simulink model "gm_model_biquad_wfa"  (R2020b)
settings: Solver=VariableStepAuto  StartTime=0.0  StopTime=1  RelTol=1e-3
undefined symbols (not defined in the file or in its folder): dfilt, in_cos, Wkn
libraries: simulink x2, dsparch4 x1
settings Model: Creator=pablo  LastModifiedBy=pablo
settings OptimizationCC: BlockReduction=off  ConditionallyExecuteInputs=off
settings DebuggingCC: ArtificialAlgebraicLoopMsg=none  InheritedTsInSrcMsg=none

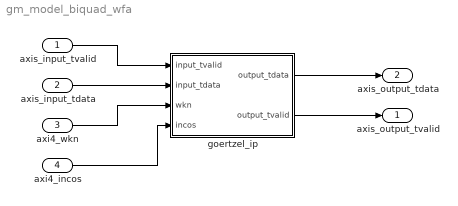
== system gm_model_biquad_wfa ==
  axis_input_tvalid : Inport  OutDataTypeStr=boolean  PortDimensions=1  SampleTime=0.001
  axis_input_tdata : Inport  Port=2  OutDataTypeStr=fixdt(1, 32, 16)  PortDimensions=1  SampleTime=0.001
  axi4_wkn : Inport  Port=3  OutDataTypeStr=fixdt(1, 32, 16)  PortDimensions=1  SampleTime=0.001
  axi4_incos : Inport  Port=4  OutDataTypeStr=fixdt(1, 32, 16)  PortDimensions=1  SampleTime=0.001
  goertzel_ip : Subsystem
  axis_output_tvalid : Outport
  axis_output_tdata : Outport  Port=2
  wires:
  axis_input_tvalid/1 -> goertzel_ip/1(input_tvalid)
  axis_input_tdata/1 -> goertzel_ip/2(input_tdata)
  axi4_wkn/1 -> goertzel_ip/3(wkn)
  axi4_incos/1 -> goertzel_ip/4(incos)
  goertzel_ip/1(output_tdata) -> axis_output_tdata/1
  goertzel_ip/2(output_tvalid) -> axis_output_tvalid/1

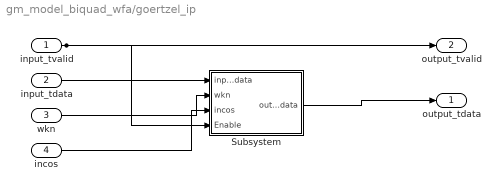
== system gm_model_biquad_wfa/goertzel_ip ==
  input_tvalid : Inport  OutDataTypeStr=boolean  PortDimensions=1  SampleTime=0.001
  input_tdata : Inport  Port=2  OutDataTypeStr=fixdt(1, 32, 16)  PortDimensions=1  SampleTime=0.001
  wkn : Inport  Port=3  OutDataTypeStr=fixdt(1, 32, 16)  PortDimensions=1  SampleTime=0.001
  incos : Inport  Port=4  OutDataTypeStr=fixdt(1, 32, 16)  PortDimensions=1  SampleTime=0.001
  Subsystem : Subsystem
  output_tdata : Outport
  output_tvalid : Outport  Port=2  InitialOutput=0
  wires:
  input_tvalid/1 -> output_tvalid/1, Subsystem/4(Enable)
  input_tdata/1 -> Subsystem/1(input_data)
  wkn/1 -> Subsystem/2(wkn)
  incos/1 -> Subsystem/3(incos)
  Subsystem/1(output_data) -> output_tdata/1

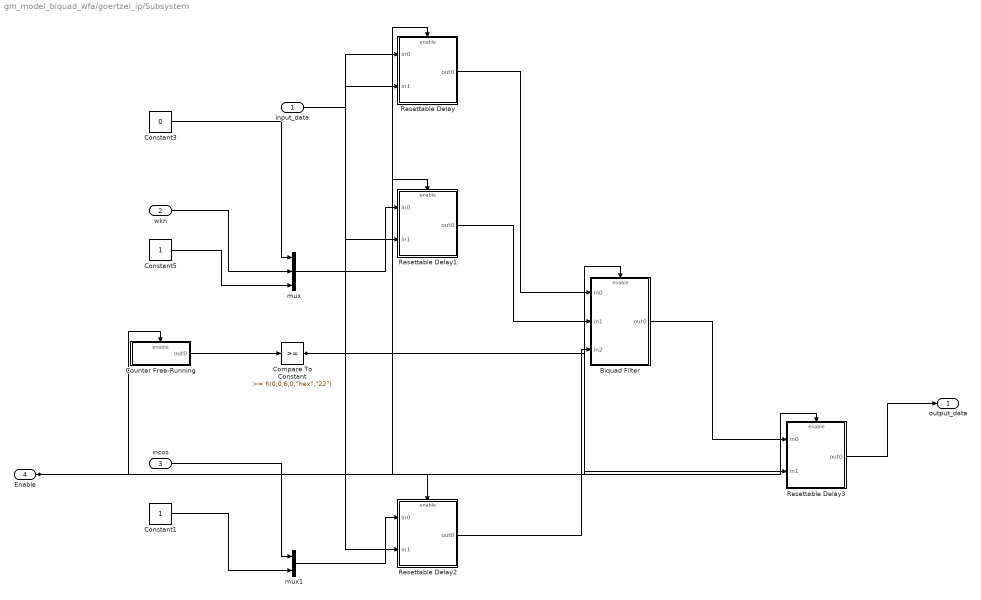
== system gm_model_biquad_wfa/goertzel_ip/Subsystem ==
  input_data : Inport  OutDataTypeStr=fixdt(1, 32, 16)  PortDimensions=1  SampleTime=0.001
  wkn : Inport  Port=2  OutDataTypeStr=fixdt(1, 32, 16)  PortDimensions=1  SampleTime=0.001
  incos : Inport  Port=3  OutDataTypeStr=fixdt(1, 32, 16)  PortDimensions=1  SampleTime=0.001
  Enable : Inport  Port=4  OutDataTypeStr=boolean  SampleTime=0.001
  Biquad Filter : Subsystem
      settings: MinAlgLoopOccurrences=on
  Compare To Constant : simulink/Logic and Bit Operations/Compare To Constant  relop=>=  const="fi(0,0,6,0,\"hex\",\"22\")"  OutDataTypeStr=boolean
  Constant1 : Constant  OutDataTypeStr=fixdt(1, 32, 16)
  Constant3 : Constant  Value=0  OutDataTypeStr=fixdt(1, 32, 16)
  Constant5 : Constant  OutDataTypeStr=fixdt(1, 32, 16)
  Counter Free-Running : Subsystem
      settings: MinAlgLoopOccurrences=on
  Resettable Delay : Subsystem
      settings: MinAlgLoopOccurrences=on
  Resettable Delay1 : Subsystem
      settings: MinAlgLoopOccurrences=on
  Resettable Delay2 : Subsystem
      settings: MinAlgLoopOccurrences=on
  Resettable Delay3 : Subsystem
      settings: MinAlgLoopOccurrences=on
  mux : Mux  Inputs=3
  mux1 : Mux  Inputs=2
  output_data : Outport  InitialOutput=0
  wires:
  Enable/1 -> Biquad Filter/Enable, Resettable Delay3/Enable, Resettable Delay2/Enable, Resettable Delay1/Enable, Resettable Delay/Enable, Counter Free-Running/Enable
  input_data/1 -> Resettable Delay/1(in0)
  wkn/1 -> mux/2
  incos/1 -> mux1/1
  Biquad Filter/1(out0) -> Resettable Delay3/1(in0)
  Compare To Constant/1 -> Resettable Delay3/2(in1), Resettable Delay2/2(in1), Resettable Delay1/2(in1), Resettable Delay/2(in1)
  Constant1/1 -> mux1/2
  Constant3/1 -> mux/1
  Constant5/1 -> mux/3
  Counter Free-Running/1(out0) -> Compare To Constant/1
  mux/1 -> Resettable Delay1/1(in0)
  mux1/1 -> Resettable Delay2/1(in0)
  Resettable Delay/1(out0) -> Biquad Filter/1(in0)
  Resettable Delay1/1(out0) -> Biquad Filter/2(in1)
  Resettable Delay2/1(out0) -> Biquad Filter/3(in2)
  Resettable Delay3/1(out0) -> output_data/1

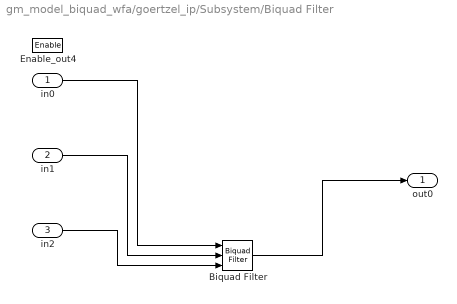
== system gm_model_biquad_wfa/goertzel_ip/Subsystem/Biquad Filter ==
  in0 : Inport  OutDataTypeStr=fixdt(1, 32, 16)  SampleTime=0.001
  in1 : Inport  Port=2  OutDataTypeStr=fixdt(1, 32, 16)  PortDimensions=[3]  SampleTime=0.001
  in2 : Inport  Port=3  OutDataTypeStr=fixdt(1, 32, 16)  PortDimensions=[2 1]  SampleTime=0.001
  Enable_out4 : EnablePort  OutDataTypeStr=boolean
  Biquad Filter : dsparch4/Biquad Filter  FilterSource=Input port(s)  CoeffSource=Specify via dialog  FilterObject=dfilt.df2tsos([1 0.3 0.4],[1 0.1 0.2])  IIRFiltStruct=Direct form II transposed  BiQuadCoeffs=[0 1 real(Wkn) 1 -in_cos 1]  ScaleValues=1  IC=0  ICnum=0  ICden=0  a0Flag=Warning  optimizeScaleValues=on  ScaleValueMode=Assume all are unity and optimize  roundingMode=Floor  overflowMode=off  scaleValueFracLength=14  denProdOutputFracLength=30  denAccumFracLength=30  secondMemoryFracLength=15
      settings: SourceProductName=DSP System Toolbox
  out0 : Outport  OutDataTypeStr=fixdt(1, 32, 16)  InitialOutput=0
  wires:
  Biquad Filter/1 -> out0/1
  in0/1 -> Biquad Filter/1
  in1/1 -> Biquad Filter/2
  in2/1 -> Biquad Filter/3

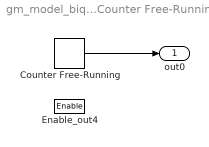
== system gm_model_biquad_wfa/goertzel_ip/Subsystem/Counter Free-Running ==
  Enable_out4 : EnablePort  OutDataTypeStr=boolean
  Counter Free-Running : simulink/Sources/Counter Free-Running  NumBits=6  tsamp=0.001
  out0 : Outport  OutDataTypeStr=fixdt(0, 6, 0)  InitialOutput=0
  wires:
  Counter Free-Running/1 -> out0/1

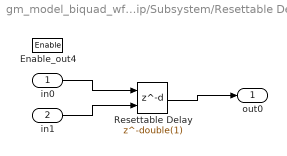
== system gm_model_biquad_wfa/goertzel_ip/Subsystem/Resettable Delay ==
  in0 : Inport  OutDataTypeStr=fixdt(1, 32, 16)  SampleTime=0.001
  in1 : Inport  Port=2  OutDataTypeStr=boolean  SampleTime=0.001
  Enable_out4 : EnablePort  OutDataTypeStr=boolean
  Resettable Delay : Delay  DelayLength=double(1)  InitialCondition="fi(0,1,32,16,\"hex\",\"00000000\")"  ExternalReset=Level
      settings: InputPortMap=u0,r5
  out0 : Outport  OutDataTypeStr=fixdt(1, 32, 16)  InitialOutput=0
  wires:
  Resettable Delay/1 -> out0/1
  in0/1 -> Resettable Delay/1
  in1/1 -> Resettable Delay/2

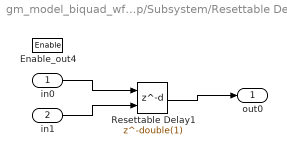
== system gm_model_biquad_wfa/goertzel_ip/Subsystem/Resettable Delay1 ==
  in0 : Inport  OutDataTypeStr=fixdt(1, 32, 16)  PortDimensions=[3]  SampleTime=0.001
  in1 : Inport  Port=2  OutDataTypeStr=boolean  SampleTime=0.001
  Enable_out4 : EnablePort  OutDataTypeStr=boolean
  Resettable Delay1 : Delay  DelayLength=double(1)  InitialCondition="fi(0,1,32,16,\"hex\",\"00000000\")"  ExternalReset=Level
      settings: InputPortMap=u0,r5
  out0 : Outport  OutDataTypeStr=fixdt(1, 32, 16)  PortDimensions=[3]  InitialOutput=0
  wires:
  Resettable Delay1/1 -> out0/1
  in0/1 -> Resettable Delay1/1
  in1/1 -> Resettable Delay1/2

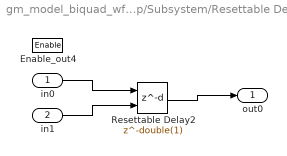
== system gm_model_biquad_wfa/goertzel_ip/Subsystem/Resettable Delay2 ==
  in0 : Inport  OutDataTypeStr=fixdt(1, 32, 16)  PortDimensions=[2 1]  SampleTime=0.001
  in1 : Inport  Port=2  OutDataTypeStr=boolean  SampleTime=0.001
  Enable_out4 : EnablePort  OutDataTypeStr=boolean
  Resettable Delay2 : Delay  DelayLength=double(1)  InitialCondition="fi(0,1,32,16,\"hex\",\"00000000\")"  ExternalReset=Level
      settings: InputPortMap=u0,r5
  out0 : Outport  OutDataTypeStr=fixdt(1, 32, 16)  PortDimensions=[2 1]  InitialOutput=0
  wires:
  Resettable Delay2/1 -> out0/1
  in0/1 -> Resettable Delay2/1
  in1/1 -> Resettable Delay2/2

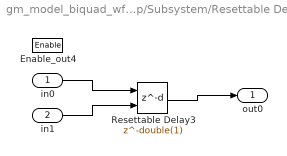
== system gm_model_biquad_wfa/goertzel_ip/Subsystem/Resettable Delay3 ==
  in0 : Inport  OutDataTypeStr=fixdt(1, 32, 16)  SampleTime=0.001
  in1 : Inport  Port=2  OutDataTypeStr=boolean  SampleTime=0.001
  Enable_out4 : EnablePort  OutDataTypeStr=boolean
  Resettable Delay3 : Delay  DelayLength=double(1)  InitialCondition="fi(0,1,32,16,\"hex\",\"00000000\")"  ExternalReset=Level
      settings: InputPortMap=u0,r5
  out0 : Outport  OutDataTypeStr=fixdt(1, 32, 16)  InitialOutput=0
  wires:
  Resettable Delay3/1 -> out0/1
  in0/1 -> Resettable Delay3/1
  in1/1 -> Resettable Delay3/2
